simulink model "aebMS"  (R2016a)
settings: Solver=FixedStepDiscrete  StartTime=0.0  StopTime=inf  FixedStep=0.1  RelTol=1e-3
libraries: frdmk64flib x2
settings Model: SimulationMode=external  ExtModeTrigDuration=5  Creator=Gaspare  LastModifiedBy=Gaspare
settings OptimizationCC: OptimizeModelRefInitCode=on  LifeSpan=1  MaxStackSize=64
settings HardwareCC: ProdBitPerPointer=32  ProdLargestAtomicInteger=Long  ProdLargestAtomicFloat=Double  ProdWordSize=32  ProdHWDeviceType=ARM Compatible->ARM Cortex
settings RTWCC: SystemTargetFile=ert.tlc  HardwareBoard=Freescale FRDM-K64F  TemplateMakefile=ert_default_tmf  GenerateReport=on  Toolchain=GNU Tools for ARM Embedded Processors  IncludeHyperlinkInReport=on  LaunchReport=on  GenerateTraceInfo=on  GenerateTraceReport=on  GenerateTraceReportSl=on  GenerateTraceReportSf=on  GenerateTraceReportEml=on
settings CodeAppCC: ForceParamTrailComments=on  IgnoreCustomStorageClasses=off  OperatorAnnotations=on  SimulinkDataObjDesc=on  SFDataObjDesc=on  MATLABFcnDesc=on  InsertBlockDesc=on  MATLABSourceComments=on
settings ERTTargetCC: ERTFilePackagingFormat=Compact

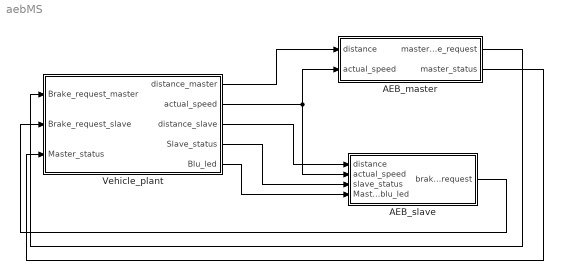
== system aebMS ==
  AEB_master : Subsystem
  AEB_slave : Subsystem
  Vehicle_plant : Subsystem
  wires:
  Vehicle_plant/1(distance_master) -> AEB_master/1(distance)
  Vehicle_plant/2(actual_speed) -> AEB_slave/2(actual_speed), AEB_master/2(actual_speed)
  AEB_slave/1(brake request) -> Vehicle_plant/2(Brake_request_slave)
  Vehicle_plant/3(distance_slave) -> AEB_slave/1(distance)
  AEB_master/1(master_brake_request) -> Vehicle_plant/1(Brake_request_master)
  AEB_master/2(master_status) -> Vehicle_plant/3(Master_status)
  Vehicle_plant/4(Slave_status) -> AEB_slave/3(slave_status)
  Vehicle_plant/5(Blu_led) -> AEB_slave/4(Masted_blu_led)

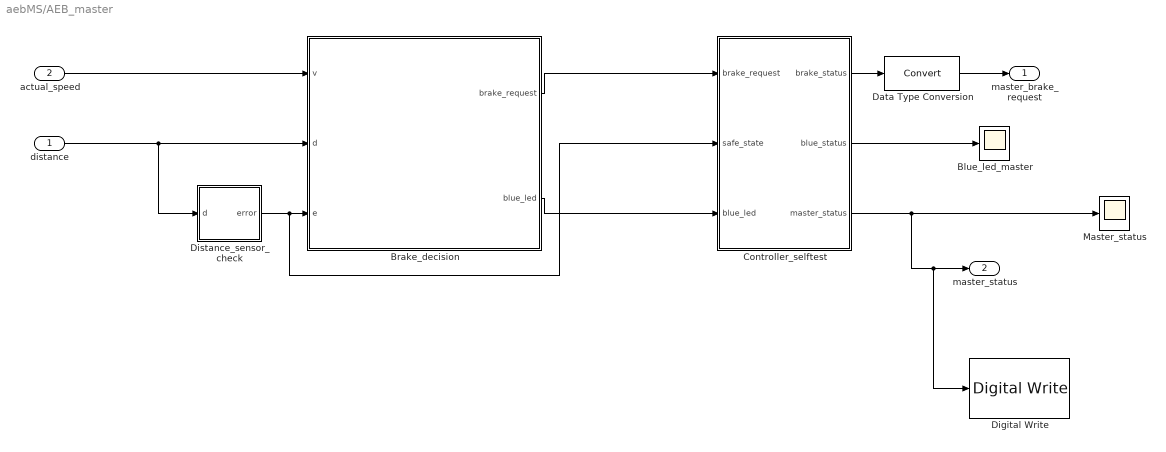
== system aebMS/AEB_master ==
  distance : Inport
  actual_speed : Inport  Port=2
  Blue_led_master : Scope
  Brake_decision : Stateflow chart  TreatAsAtomicUnit=on
  Controller_selftest : Stateflow chart  TreatAsAtomicUnit=on
  Data Type Conversion : DataTypeConversion
  Digital Write : frdmk64flib/Digital Write  Whichpin=RED_LED
  Distance_sensor_check : Stateflow chart  TreatAsAtomicUnit=on
  Master_status : Scope
  master_brake_request : Outport
  master_status : Outport  Port=2
  wires:
  actual_speed/1 -> Brake_decision/1(v)
  distance/1 -> Distance_sensor_check/1(d), Brake_decision/2(d)
  Brake_decision/1(brake_request) -> Controller_selftest/1(brake_request)
  Brake_decision/2(blue_led) -> Controller_selftest/3(blue_led)
  Controller_selftest/2(blue_status) -> Blue_led_master/1
  Controller_selftest/1(brake_status) -> Data Type Conversion/1
  Distance_sensor_check/1(error) -> Controller_selftest/2(safe_state), Brake_decision/3(e)
  Controller_selftest/3(master_status) -> Digital Write/1, master_status/1, Master_status/1
  Data Type Conversion/1 -> master_brake_request/1

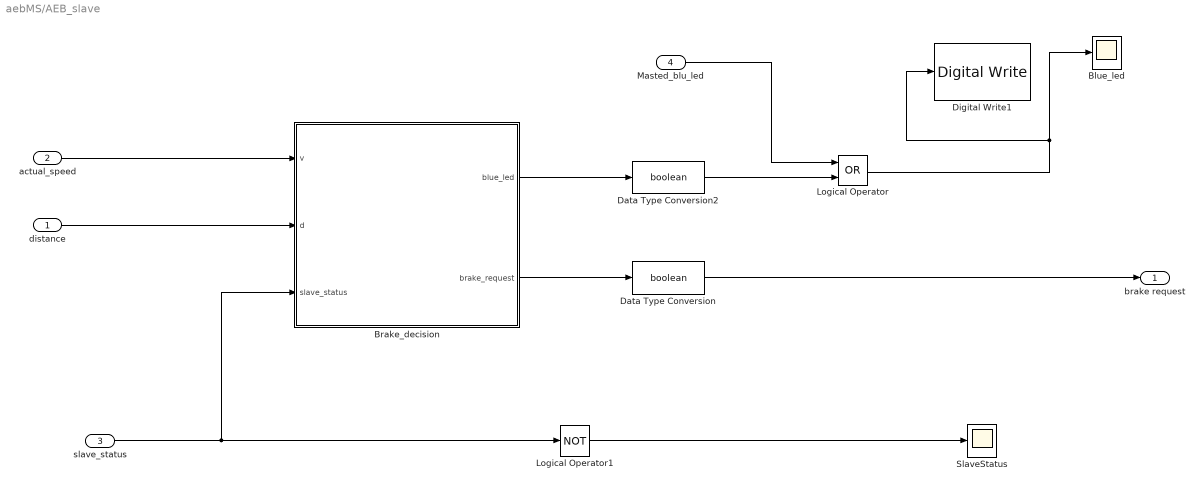
== system aebMS/AEB_slave ==
  distance : Inport
  actual_speed : Inport  Port=2
  slave_status : Inport  Port=3
  Masted_blu_led : Inport  Port=4
  Blue_led : Scope
  Brake_decision : Stateflow chart  TreatAsAtomicUnit=on
  Data Type Conversion : DataTypeConversion  OutDataTypeStr=boolean
  Data Type Conversion2 : DataTypeConversion  OutDataTypeStr=boolean
  Digital Write1 : frdmk64flib/Digital Write  Whichpin=BLUE_LED
  Logical Operator : Logic  Operator=OR  AllPortsSameDT=off  OutDataTypeStr=boolean
  Logical Operator1 : Logic  Operator=NOT  AllPortsSameDT=off  OutDataTypeStr=boolean
  SlaveStatus : Scope
  brake request : Outport  OutDataTypeStr=boolean
  wires:
  Logical Operator/1 -> Blue_led/1, Digital Write1/1
  Brake_decision/1(blue_led) -> Data Type Conversion2/1
  Brake_decision/2(brake_request) -> Data Type Conversion/1
  distance/1 -> Brake_decision/2(d)
  actual_speed/1 -> Brake_decision/1(v)
  Data Type Conversion/1 -> brake request/1
  slave_status/1 -> Brake_decision/3(slave_status), Logical Operator1/1
  Data Type Conversion2/1 -> Logical Operator/2
  Masted_blu_led/1 -> Logical Operator/1
  Logical Operator1/1 -> SlaveStatus/1

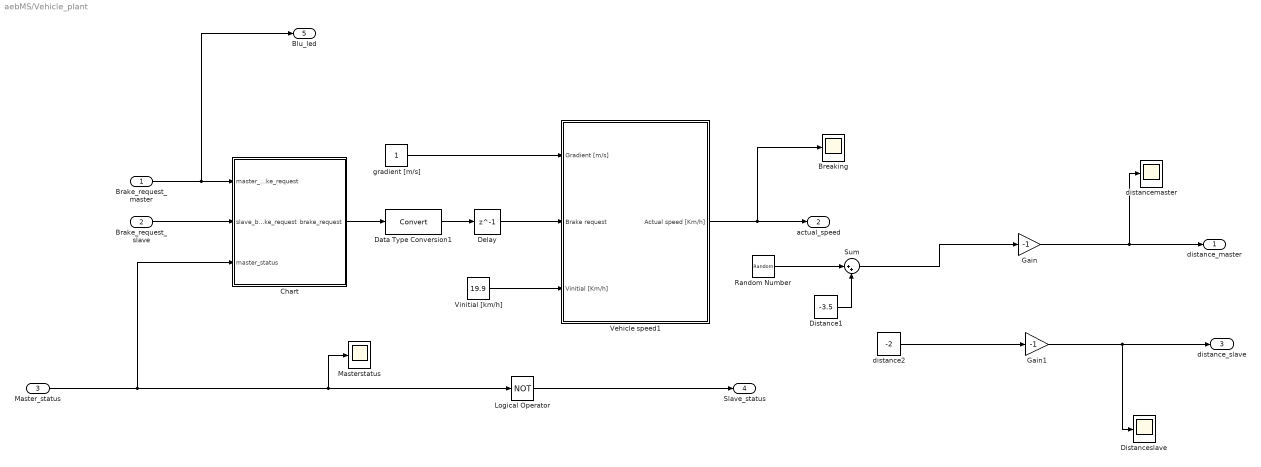
== system aebMS/Vehicle_plant ==
  Brake_request_master : Inport  OutDataTypeStr=boolean
  Brake_request_slave : Inport  Port=2
  Master_status : Inport  Port=3
  Breaking : Scope
  Chart : Stateflow chart  TreatAsAtomicUnit=on
  Data Type Conversion1 : DataTypeConversion
  Delay : Delay  DelayLength=1  InitialCondition=0
  Distance1 : Constant  Value=-3.5
  Distanceslave : Scope
  Gain : Gain  Gain=-1
  Gain1 : Gain  Gain=-1
  Logical Operator : Logic  Operator=NOT  AllPortsSameDT=off  OutDataTypeStr=boolean
  Masterstatus : Scope
  Random Number : RandomNumber  Mean=0.5  Variance=.5  SampleTime=0.1
  Sum : Sum  Inputs=|++
  Vehicle speed1 : Subsystem
  Vinitial [km/h] : Constant  Value=19.9
  distance2 : Constant  Value=-2
  distancemaster : Scope
  gradient [m/s] : Constant
  distance_master : Outport
  actual_speed : Outport  Port=2
  distance_slave : Outport  Port=3
  Slave_status : Outport  Port=4
  Blu_led : Outport  Port=5
  wires:
  gradient [m/s]/1 -> Vehicle speed1/1(Gradient [m/s])
  Vinitial [km/h]/1 -> Vehicle speed1/3(Vinitial [Km/h])
  Vehicle speed1/1(Actual speed [Km/h]) -> Breaking/1, actual_speed/1
  Gain/1 -> distancemaster/1, distance_master/1
  Delay/1 -> Vehicle speed1/2(Brake request)
  Data Type Conversion1/1 -> Delay/1
  Gain1/1 -> distance_slave/1, Distanceslave/1
  distance2/1 -> Gain1/1
  Brake_request_master/1 -> Blu_led/1, Chart/1(master_brake_request)
  Brake_request_slave/1 -> Chart/2(slave_brake_request)
  Master_status/1 -> Masterstatus/1, Logical Operator/1, Chart/3(master_status)
  Chart/1(brake_request) -> Data Type Conversion1/1
  Logical Operator/1 -> Slave_status/1
  Distance1/1 -> Sum/2
  Sum/1 -> Gain/1
  Random Number/1 -> Sum/1

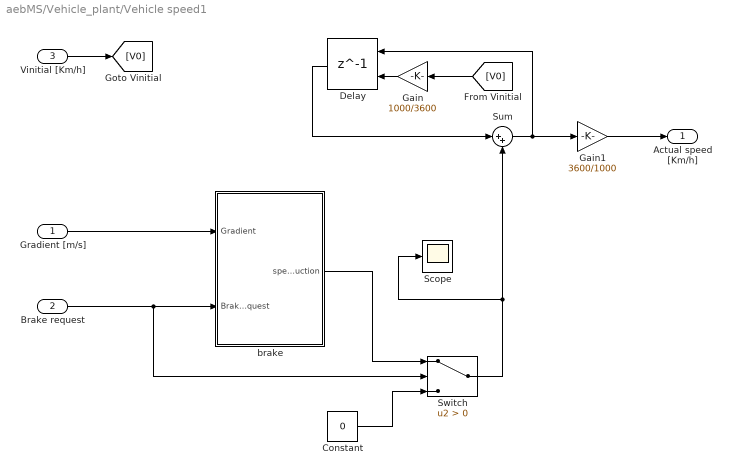
== system aebMS/Vehicle_plant/Vehicle speed1 ==
  Gradient [m/s] : Inport
  Brake request : Inport  Port=2
  Vinitial [Km/h] : Inport  Port=3
  Constant : Constant  Value=0
  Delay : Delay  DelayLength=1  InitialConditionSource=Input port  InitialCondition=0
      settings: InputPortMap=u0,p4
  Gain : Gain  Gain=1000/3600
  Gain1 : Gain  Gain=3600/1000
  Scope : Scope
  Sum : Sum  Inputs=|++
  Switch : Switch  Criteria=u2 > Threshold
  brake : Subsystem
  Actual speed [Km/h] : Outport
  wires:
  Brake request/1 -> Switch/2, brake/2(Brake request)
  Gradient [m/s]/1 -> brake/1(Gradient)
  Gain/1 -> Delay/2
  Gain1/1 -> Actual speed [Km/h]/1
  Sum/1 -> Gain1/1, Delay/1
  [V0] -> Gain/1
  Delay/1 -> Sum/1
  Vinitial [Km/h]/1 -> [V0]
  brake/1(speed_reduction) -> Switch/1
  Switch/1 -> Sum/2, Scope/1
  Constant/1 -> Switch/3

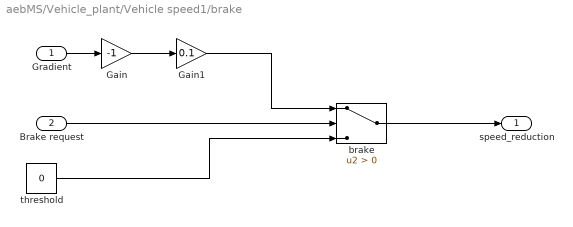
== system aebMS/Vehicle_plant/Vehicle speed1/brake ==
  Gradient : Inport
  Brake request : Inport  Port=2
  Gain : Gain  Gain=-1
  Gain1 : Gain  Gain=0.1
  brake : Switch  Criteria=u2 > Threshold
  threshold : Constant  Value=0
  speed_reduction : Outport
  wires:
  Gain/1 -> Gain1/1
  Gradient/1 -> Gain/1
  Gain1/1 -> brake/1
  Brake request/1 -> brake/2
  threshold/1 -> brake/3
  brake/1 -> speed_reduction/1

== stateflow chart aebMS/AEB_master/Distance_sensor_check ==
  state No_errors
    en:
    error=0;
  state Yes_errors
    en:
    error=1;
  (default) -> No_errors
  No_errors -> Yes_errors : [d<0.02||d>4]
  data: d input; error output

== stateflow chart aebMS/AEB_master/Controller_selftest ==
  state controller_ok
    en,du:
    brake_status=brake_request;
    master_status=safe_state;
    blue_status=blue_led;
  state controller_ko
    en,du:
    master_status=1;
    blue_status=0;
    brake_status=0;
  (default) -> controller_ok
  controller_ok -> controller_ko : [ (((brake_status==1&&master_status==0&&blue_status==1))||((brake_status==0&&blue_status==0))||((master_status==0&&blue_status==0&&brake_status==0)))~=1]
  data: brake_request input; safe_state input; blue_led input; brake_status output; blue_status output; master_status output

== stateflow chart aebMS/AEB_master/Brake_decision ==
  state No_brake
    en:
    brake_request= 0;
    blue_led=0;
  state brake
    en:
    brake_request= 1;
    blue_led=1
  (default) -> No_brake
  brake -> No_brake : [v*v*0.01< d || e==1]
  No_brake -> brake : [v*v*0.01>= d && e==0]
  data: v input; brake_request output; d input; e input; blue_led output

== stateflow chart aebMS/AEB_slave/Brake_decision ==
  state No_brake
    en:
    brake_request= 0;
    blue_led=0;
  state brake
    en:
    brake_request= 1;
    blue_led=1
  (default) -> No_brake
  brake -> No_brake : [v*v*0.01< d||slave_status==1 ]
  No_brake -> brake : [v*v*0.01>= d&&slave_status==0&&(d>0.02||d<4)]
  data: blue_led output; v input; brake_request output; d input; slave_status input

== stateflow chart aebMS/Vehicle_plant/Chart ==
  state master_ok
    du:
    brake_request=master_brake_request;
  state master_ko
    du:
    brake_request=slave_brake_request;
  (default) -> master_ok
  master_ok -> master_ko : [master_status==1]
  data: master_brake_request input; slave_brake_request input; master_status input; brake_request output
